simulink model "SimulinkOnrampProjectFalconpart1"  (R2019b)
settings: Solver=VariableStepAuto  StartTime=0.0  StopTime=10.0  RelTol=1e-3
StartFcn:
  | learning.simulink.clearGlows(gcs);learning.simulink.resetGraderBadge(gcs);learning.simulink.closeNotificationBar(gcs);learning.simulink.Application.getInstance().clearStateflowBreakpoints()
StopFcn:
  | save_system(gcs);learning.simulink.refreshSignalWindows
model workspace (MAT data in the model file):
  courseObject.course = 'simulink'
  courseObject.chapter = 13
  courseObject.lesson = 1
  courseObject.section = 2
  courseObject.task = 1
  t_ans = [0; 0.1; 0.2; 0.3; 0.4; 0.5; 0.6; 0.7; 0.8; 0.9; 1; 1.1; 1.2; 1.3; 1.4; 1.5; 1.6; 1.7; 1.8; 1.9; 2; 2.1; 2.2; 2.3; 2.4; 2.5; 2.6; 2.7; 2.8; 2.9; 3; 3.1; 3.2; 3.3; 3.4; 3.5; 3.6; 3.7; 3.8; 3.9; 4; 4.1; 4.2; 4.3; 4.4; 4.5; 4.6; 4.7; 4.8; 4.9; 5; 5.1; 5.2; 5.3; 5.4; 5.5; 5.6; 5.7; 5.8; 5.9; 6; 6.1; 6.2; 6.3; 6.4; 6.5; 6.6; 6.7; 6.8; 6.9; 7; 7.1; 7.2; 7.3; 7.4; 7.5; 7.6; 7.7; 7.8; 7.9; 8; 8.1; 8.2; 8.3; 8.4; 8.5; 8.6; 8.7; 8.8; 8.9; 9; 9.1; 9.2; 9.3; 9.4; 9.5; 9.6; 9.7; 9.8; 9.9; 10]
  y_ans = [0; -0.000200950914521; -0.00120570548708; -0.00622947834396; -0.0313483418766; -0.156942565284; -0.784901893294; -1.76577331462; -2.7463838085; -3.72658860853; -4.70624318793; -5.68520334466; -6.66332528615; -7.6404657135; -8.61648190506; -9.59123179932; -10.5645740769; -11.5363682419; -12.5064747015; -13.4747548455; -14.441071124; -15.4052871236; -16.3672676426; -17.3268787648; -18.2839879315; -19.2384640119; -20.1901773717; -21.1389999403; -22.0848052757; -23.0274686279; -23.9668669998; -24.9028792065; -25.8353859326; -26.7642697869; -27.6894153551; -28.6107092507; -29.5280401631; -30.4412989032; -31.3503784479; -32.2551739806; -33.155582931; -34.0515050107; -34.9428422483; -35.8294990206; -36.7113820823; -37.5884005928; -38.4604661409; -39.3274927668; -40.1893969821; -41.0460977871; -41.897516686; -42.7435776993; -43.5842073747; -44.4193347949; -45.2488915838; -46.07281191; -46.8910324884; -47.7034925794; -48.5101339867; -49.3109010518; -50.1057406481; -50.8946021713; -51.6774375295; -52.4542011303; -53.2248498666; -53.9893431006; -54.7476426461; -55.4997127492; -56.245520067; -56.9850336459; -57.7182248966; -58.44506757; -59.1655377296; -59.8796137241; -60.587276158; -61.2885078616; -61.9832938595; -62.6716213379; -63.3534796118; -64.0288600902; -64.6977562414; -65.3601635567; -66.0160795141; -66.6655035409; -67.3084369754; -67.944883029; -68.574846747; -69.1983349691; -69.8153562894; -70.4259210168; -71.0300411339; -71.627730257; -72.2190035946; -72.8038779066; -73.3823714634; -73.9545040045; -74.5202966974; -75.0797720963; -75.6329541014; -76.1798679174; -76.7205400132; -77.2549980811; -77.7832709962; -78.3053887764; -78.8213825426; -79.3312844789; -79.4324778498]
  y_ans2 = [-10; -10.9727094721; -11.9438121188; -12.9131687504; -13.8806411923; -14.8460923624; -15.8093863468; -16.7703884748; -17.7289653912; -18.6849851282; -19.638317175; -20.5888325457; -21.5364038454; -22.4809053349; -23.4222129926; -24.3602045751; -25.2947596755; -26.2257597794; -27.1530883193; -28.0766307262; -28.996274479; -29.9119091523; -30.8234264612; -31.7307203038; -32.6336868018; -33.5322243386; -34.4262335943; -35.3156175796; -36.200281666; -37.0801336145; -37.9550836015; -38.8250442421; -39.6899306119; -40.5496602652; -41.4041532515; -42.2533321299; -43.0971219808; -43.9354504151; -44.7682475816; -45.5954461721; -46.416981424; -47.2327911211; -48.0428155916; -48.8469977055; -49.6452828679; -50.4376190122; -51.2239565902; -52.0042485608; -52.7784503768; -53.5465199696; -54.308417733; -55.064106504; -55.8135515436; -56.5567205147; -57.2935834591; -58.0241127731; -58.7482831816; -59.4660717109; -60.1774576603; -60.8824225724; -61.5809502024; -62.2730264864; -62.9586395083; -63.6377794663; -64.3104386383; -64.9766113461; -65.6362939195; -66.2894846594; -66.9361837999; -67.5763934704; -68.2101176569; -68.8373621626; -69.4581345686; -70.0724441939; -70.6803020548; -71.2817208247; -71.8767147932; -72.4652998251; -73.0474933194; -73.6233141681; -74.1927827153; -74.7559207156; -75.3127512931; -75.8632989006; -76.4075892786; -76.9456494144; -77.4775075017; -78.0031929002; -78.5227360957; -79.0361686602; -79.5435232125; -80.0448333792; -80.5401337561; -81.0294598695; -81.5128481389; -81.9903358391; -82.4619610636; -82.9277626878; -83.3877803336; -83.8420543333; -84.2906256952]
undefined symbols (not defined in the file): A, Cd, g, m, rho
CloseFcn:
  | learning.simulink.cleanupOnlineTraining
settings Model: Creator=sahil  LastModifiedBy=sahil
settings DataIOCC: SaveTime=off

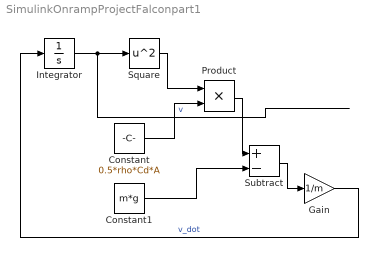
== system SimulinkOnrampProjectFalconpart1 ==
  Constant : Constant  Value=0.5*rho*Cd*A
  Constant1 : Constant  Value=m*g
  Gain : Gain  Gain=1/m
  Integrator : Integrator  InitialCondition=-10
  Product : Product
  Square : Math  Operator=square  SignedPower=off  SaturateOnIntegerOverflow=on
  Subtract : Sum  Inputs=+-
  wires:
  Gain/1 -> Integrator/1  "v_dot"
  Integrator/1 -> Square/1  "v"
  Constant/1 -> Product/2
  Square/1 -> Product/1
  Subtract/1 -> Gain/1
  Constant1/1 -> Subtract/2
  Product/1 -> Subtract/1
